simulink model "FOC"  (R2024b)
settings: Solver=VariableStepAuto  StartTime=0.0  StopTime=10.0  RelTol=1e-3
undefined symbols (not defined in the file): U
settings Model: SimulationMode=accelerator  Creator=misaka10039  LastModifiedBy=changeo

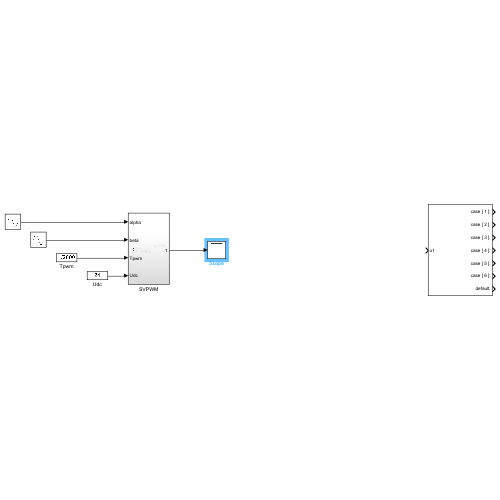
[thumbnail: Simulink's stored preview of the top-level diagram]
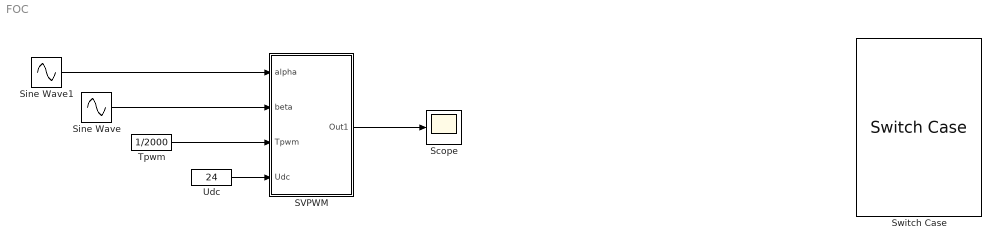
== system FOC ==
  SVPWM : Subsystem
  Scope : Scope
  Sine Wave : Sin  Frequency=pi  SampleTime=0
  Sine Wave1 : Sin  Frequency=pi  Phase=pi/2  SampleTime=0
  Switch Case : SwitchCase  CaseConditions={1,2,3,4,5,6}
  Tpwm : Constant  Value=1/2000
  Udc : Constant  Value=24
  wires:
  Sine Wave1/1 -> SVPWM/1(alpha)
  Sine Wave/1 -> SVPWM/2(beta)
  SVPWM/1(Out1) -> Scope/1
  Tpwm/1 -> SVPWM/3(Tpwm)
  Udc/1 -> SVPWM/4(Udc)

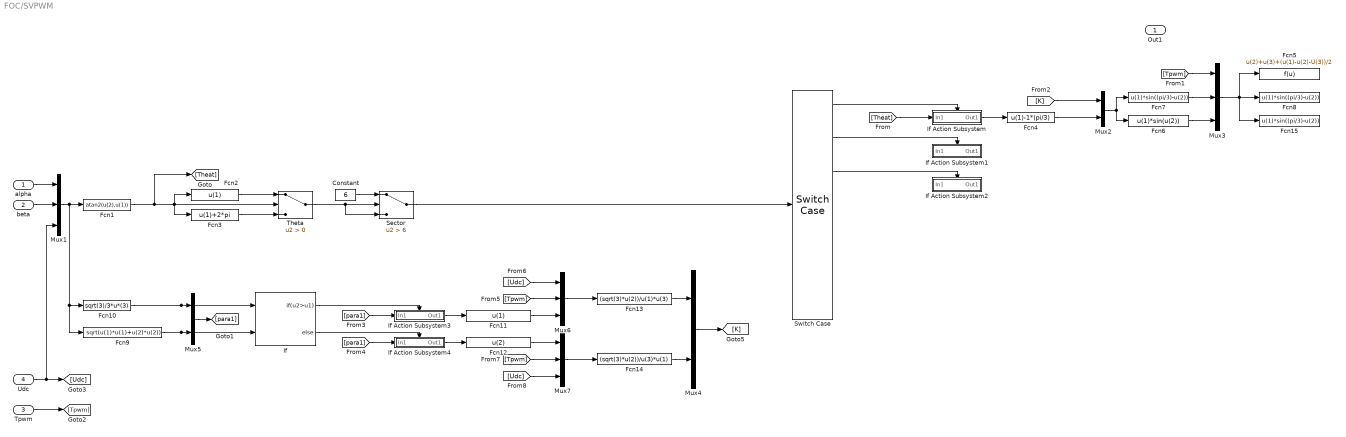
== system FOC/SVPWM ==
  alpha : Inport
  beta : Inport  Port=2
  Tpwm : Inport  Port=3
  Udc : Inport  Port=4
  Constant : Constant  Value=6
  Fcn1 : Fcn  Expr=atan2(u(2),u(1))
  Fcn10 : Fcn  Expr=sqrt(3)/3*u*(3)
  Fcn11 : Fcn  Expr=u(1)
  Fcn12 : Fcn  Expr=u(2)
  Fcn13 : Fcn  Expr=(sqrt(3)*u(2))/u(1)*u(3)
  Fcn14 : Fcn  Expr=(sqrt(3)*u(2))/u(3)*u(1)
  Fcn15 : Fcn  Expr=u(1)*sin((pi/3)-u(2))
  Fcn2 : Fcn  Expr=u(1)
  Fcn3 : Fcn  Expr=u(1)+2*pi
  Fcn4 : Fcn  Expr=u(1)-1*(pi/3)
  Fcn5 : Fcn  Expr=u(2)+u(3)+(u(1)-u(2)-U(3))/2
  Fcn6 : Fcn  Expr=u(1)*sin(u(2))
  Fcn7 : Fcn  Expr=u(1)*sin((pi/3)-u(2))
  Fcn8 : Fcn  Expr=u(1)*sin((pi/3)-u(2))
  Fcn9 : Fcn  Expr=sqrt(u(1)*u(1)+u(2)*u(2))
  If : If  NumInputs=2  IfExpression=u2>u1
  If Action Subsystem : Subsystem  TreatAsAtomicUnit=on
  If Action Subsystem1 : Subsystem  TreatAsAtomicUnit=on
  If Action Subsystem2 : Subsystem  TreatAsAtomicUnit=on
  If Action Subsystem3 : Subsystem  TreatAsAtomicUnit=on
  If Action Subsystem4 : Subsystem  TreatAsAtomicUnit=on
  Mux{1,3,6..7} (4 alike) : Mux  Inputs=3
  Mux2 : Mux  Inputs=2
  Mux4 : Mux  Inputs=2
  Mux5 : Mux  Inputs=2
  Sector : Switch  Criteria=u2 > Threshold  Threshold=6  SaturateOnIntegerOverflow=off  InputSameDT=off
  Switch Case : SwitchCase  CaseConditions={1,2,3,4,5,6}
  Theta : Switch  Criteria=u2 > Threshold  SaturateOnIntegerOverflow=off  InputSameDT=off
  Out1 : Outport
  wires:
  alpha/1 -> Mux1/1
  beta/1 -> Mux1/2
  Fcn1/1 -> [Theat], Fcn2/1, Fcn3/1, Theta/2
  Fcn3/1 -> Theta/3
  Fcn2/1 -> Theta/1
  Constant/1 -> Sector/1
  Sector/1 -> Switch Case/1
  Theta/1 -> Sector/3, Sector/2
  Switch Case/1 -> If Action Subsystem/Action
  Switch Case/2 -> If Action Subsystem1/Action
  Switch Case/3 -> If Action Subsystem2/Action
  If Action Subsystem/1(Out1) -> Fcn4/1
  [Theat] -> If Action Subsystem/1(In1)
  Mux2/1 -> Fcn6/1, Fcn7/1
  [K] -> Mux2/1
  Udc/1 -> [Udc], Mux1/3
  Mux1/1 -> Fcn9/1, Fcn10/1, Fcn1/1
  If/1 -> If Action Subsystem3/Action
  If/2 -> If Action Subsystem4/Action
  [para1] -> If Action Subsystem3/1(In1)
  [para1] -> If Action Subsystem4/1(In1)
  Tpwm/1 -> [Tpwm]
  Fcn9/1 -> If/2, Mux5/2
  Fcn10/1 -> If/1, Mux5/1
  Mux5/1 -> [para1]
  If Action Subsystem3/1(Out1) -> Fcn11/1
  If Action Subsystem4/1(Out1) -> Fcn12/1
  Mux6/1 -> Fcn13/1
  Fcn11/1 -> Mux6/3
  [Tpwm] -> Mux6/2
  [Udc] -> Mux6/1
  Fcn12/1 -> Mux7/1
  [Udc] -> Mux7/3
  [Tpwm] -> Mux7/2
  Mux7/1 -> Fcn14/1
  Fcn13/1 -> Mux4/1
  Fcn14/1 -> Mux4/2
  Mux4/1 -> [K]
  Fcn4/1 -> Mux2/2
  Fcn7/1 -> Mux3/2
  Fcn6/1 -> Mux3/3
  [Tpwm] -> Mux3/1
  Mux3/1 -> Fcn5/1, Fcn8/1, Fcn15/1

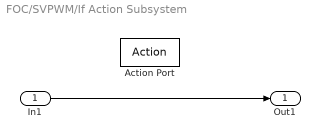
== system FOC/SVPWM/If Action Subsystem ==
  In1 : Inport
  Action Port : ActionPort  ActionPortLabel=case [ 1 ]:
  Out1 : Outport
  wires:
  In1/1 -> Out1/1

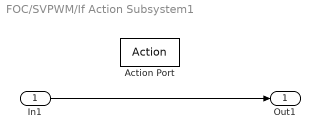
== system FOC/SVPWM/If Action Subsystem1 ==
  In1 : Inport
  Action Port : ActionPort  ActionPortLabel=case [ 2 ]:
  Out1 : Outport
  wires:
  In1/1 -> Out1/1

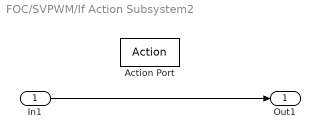
== system FOC/SVPWM/If Action Subsystem2 ==
  In1 : Inport
  Action Port : ActionPort  ActionPortLabel=case [ 3 ]:
  Out1 : Outport
  wires:
  In1/1 -> Out1/1

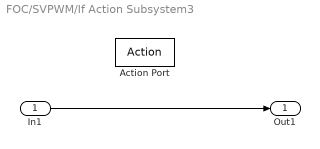
== system FOC/SVPWM/If Action Subsystem3 ==
  In1 : Inport
  Action Port : ActionPort  ActionPortLabel=if(u2>u1)
  Out1 : Outport
  wires:
  In1/1 -> Out1/1

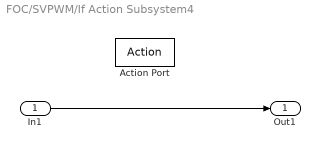
== system FOC/SVPWM/If Action Subsystem4 ==
  In1 : Inport
  Action Port : ActionPort  ActionPortLabel=else
  Out1 : Outport
  wires:
  In1/1 -> Out1/1
